simulink model "ES249A_MotAgCorrln"  (R2013b)
settings: Solver=FixedStepDiscrete  SolverMode=SingleTasking  StartTime=0.0  StopTime=1  FixedStep=0.002  RelTol=1e-3
undefined symbols (not defined in the file): FLTINJ_MOTAGCORRLN_MOTAGIDPTSIG, HALFREV_MOTREV_U0P16, MOTAGACORRLNST_CNT_U08, MotAgAMotAgBCorrln, MotAgAMotAgCCorrln, MOTAGBCORRLNST_CNT_U08, MotAgBMotAgCCorrln, MOTAGCCORRLNST_CNT_U08, MOTAGCORRLNERRTHD_MOTREVELEC_U0P16, MOTAGCORRLNNTCFAILSTEP_CNT_U16, MOTAGCORRLNNTCPASSSTEP_CNT_U16, MOTAGMAXSTALLCNTR_CNT_U08, MotAgMeclCorrlnSt, MotAgMeclIdptSig, NtcSts1, sigbuilder_block, SysGlbPrmMotPoleCnt
libraries: simulink x5
(part 2 of 4)

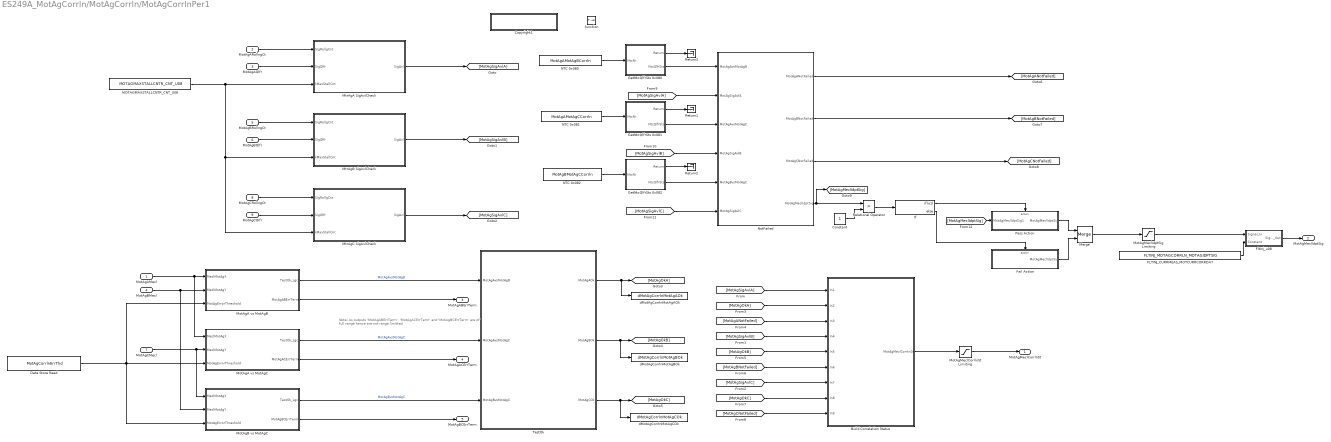
== system ES249A_MotAgCorrln/MotAgCorrln/MotAgCorrlnPer1 ==
  note: Note: As outputs 'MotAgABErrTerm', 'MotAgACErrTerm' and 'MotAgBCErrTerm'
      | are of full range hence are not range limitted
  MotAgAMecl : Inport  RequirementInfo={} %GIDa_0d510189_b4be_492d_be7e_b68d691b2df9
  MotAgARollngCt : Inport  RequirementInfo={} %GIDa_517e33a2_5a75_4f61_8f0f_573ac68cba90  Port=2
  MotAgAQlfr : Inport  RequirementInfo={} %GIDa_72867f98_7693_466f_aee4_0d6354195f1e  Port=3
  MotAgBMecl : Inport  RequirementInfo={} %GIDa_cfbccf8f_533e_4f37_986a_e6dac4ce98be  Port=4
  MotAgBRollngCt : Inport  RequirementInfo={} %GIDa_0bfa8ef6_2836_4615_abbf_8888cb320397  Port=5
  MotAgBQlfr : Inport  RequirementInfo={} %GIDa_efd6d5fa_412f_4474_a057_389b850e160a  Port=6
  MotAgCMecl : Inport  RequirementInfo={} %GIDa_b4666b4a_7a72_490a_9a26_ab5605674f7c  Port=7
  MotAgCRollngCt : Inport  RequirementInfo={} %GIDa_2a959797_a597_4b9a_b225_8bb1363b4372  Port=8
  MotAgCQlfr : Inport  RequirementInfo={} %GIDa_ae78480a_19b1_4014_b9a6_e3ccb226d53e  Port=9
  function : TriggerPort  RequirementInfo={'linktype_rmi_doors' '0000c47a (/E-STEER Core/SubSystem Specifications/Electrical Actuator/Control Module/FDD Module Requirements/EA4/ES249A_MotAgCorrln DRAFT)' '#ES249A_25' 'true' 'REQ: ES249A_25' '' ; 'linktype_rmi_doors' '0000c47a (/E-STEER Core/SubSystem Specifications/Electrical Actuator/Control Module/FDD Module Requirements/EA4/ES249A_MotAgCorrln DRAFT)' '#ES249A_76' 'true' 'REQ: ES249A_76' '' ; 'linktype_rmi_doors' '0000c47a (/E-STEER Core/SubSystem Specifications/Electrical Actuator/Control Module/FDD Module Requirements/EA4/ES249A_MotAgCorrln DRAFT)' '#ES249A_85' 'true' 'REQ: ES249A_85' '' } %GIDa_31db59e0_dbe3_46c8_b533_8d5601b81075  TriggerType=function-call
  Build Correlation Status : Subsystem  RequirementInfo={'linktype_rmi_doors' '0000c47a (/E-STEER Core/SubSystem Specifications/Electrical Actuator/Control Module/FDD Module Requirements/EA4/ES249A_MotAgCorrln DRAFT)' '#ES249A_90' 'true' 'REQ: ES249A_90' '' } %GIDa_aeadb70c_103d_495b_a56d_3da9c7a106e3
  Constant : Constant  RequirementInfo={'linktype_rmi_doors' '0000c47a (/E-STEER Core/SubSystem Specifications/Electrical Actuator/Control Module/FDD Module Requirements/EA4/ES249A_MotAgCorrln)' '#ES249A_110' 'true' 'REQ: ES249A_110' '' } %GIDa_5d96b250_1bd1_40e8_b31a_35961645f040  OutDataTypeStr=uint8
      settings: AttributesFormatString=%<OutDataTypeStr>
  Copyright1 : Subsystem  Description=|  RequirementInfo={} %GIDa_7b6edb4a_3f39_48e0_befb_44ef32e9295a  mask(Copyright Information){none=on}
      | Copyright info block.                                               
      |                                                                     
      | Place copyright information at the top of every subsystem in design.
      mask prompts: none "No parameters"
      mask help: Place copyright information at the top of every subsystem in design.
      mask Display:
      | NxtrConf = 'Nexteer Confidential';
      | 
      | sys = bdroot; %handle for the current model ("system")
      | first = get_param(sys,'Created');
      | if(isempty(first))
      |     first = datestr(now,'yyyy');
      | else
      |     first = first(end-3:end);  %year is last four digits
      | end
      | 
      | last = get_param(sys,'LastModifiedDate');
      | if isempty(last)
      |     last = datestr(now,'yyyy');
      | else
      |     last = last(end-3:end);
      | end
      | 
      | if strcmp(first,last)
      |     fprintf('%s\nCopyright  %s Nexteer',NxtrConf,first);
      | else
      |     fprintf('%s\n%s%s-%s Nexteer',NxtrConf,char(169),first,last);
      | end
  Data Store Read : DataStoreRead  DataStoreName=MotAgCorrlnErrThd
  FLTINJ_CURRMEAS_MOTCURRCORRDA7 : Constant  Value=FLTINJ_MOTAGCORRLN_MOTAGIDPTSIG
  "Fail Action " : Subsystem  RequirementInfo={'linktype_rmi_doors' '0000c47a (/E-STEER Core/SubSystem Specifications/Electrical Actuator/Control Module/FDD Module Requirements/EA4/ES249A_MotAgCorrln)' '#ES249A_110' 'true' 'REQ: ES249A_110' '' } %GIDa_4e6cbac2_25f9_4a00_a650_a831ef320943  TreatAsAtomicUnit=on
  "FltInj_u08 " : Subsystem  RequirementInfo={'linktype_rmi_doors' '0000c47a (/E-STEER Core/SubSystem Specifications/Electrical Actuator/Control Module/FDD Module Requirements/EA4/ES249A_MotAgCorrln)' '#ES249A_106' 'true' 'REQ: ES249A_106' '' } %GIDa_071c3215_62aa_4359_8caf_75f09dd6c30e  TreatAsAtomicUnit=on  VariantControl=FltInj_sim  mask(Fault_Injection){}
      mask help: Fault Injection is a simulation only block for EA3 programs.
  "GetNtcQlfrSts 0x080 " : Subsystem  RequirementInfo={'linktype_rmi_doors' '0000c47a (/E-STEER Core/SubSystem Specifications/Electrical Actuator/Control Module/FDD Module Requirements/EA4/ES249A_MotAgCorrln DRAFT)' '#ES249A_92' 'true' 'REQ: ES249A_92' '' ; 'linktype_rmi_doors' '0000c47a (/E-STEER Core/SubSystem Specifications/Electrical Actuator/Control Module/FDD Module Requirements/EA4/ES249A_MotAgCorrln DRAFT)' '#ES249A_96' 'true' 'REQ: ES249A_96' '' ; 'linktype_rmi_doors' '0000c47a (/E-STEER Core/SubSystem Specifications/Electrical Actuator/Control Module/FDD Module Requirements/EA4/ES249A_MotAgCorrln DRAFT)' '#ES249A_101' 'true' 'REQ: ES249A_101' '' ; 'linktype_rmi_doors' '0000c47a (/E-STEER Core/SubSystem Specifications/Electrical Actuator/Control Module/FDD Module Requirements/EA4/ES249A_MotAgCorrln DRAFT)' '#ES249A_102' 'true' 'REQ: ES249A_102' '' ; 'linktype_rmi_doors' '0000c47a (/E-STEER Core/SubSystem Specifications/Electrical Actuator/Control Module/FDD Module Requirements/EA4/ES249A_MotAgCorrln DRAFT)' '#ES249A_103' 'true' 'REQ: ES249A_103' '' ; 'linktype_rmi_doors' '0000c47a (/E-STEER Core/SubSystem Specifications/Electrical Actuator/Control Module/FDD Module Requirements/EA4/ES249A_MotAgCorrln DRAFT)' '#ES249A_97' 'true' 'REQ: ES249A_97' '' ; 'linktype_rmi_doors' '0000c47a (/E-STEER Core/SubSystem Specifications/Electrical Actuator/Control Module/FDD Module Requirements/EA4/ES249A_MotAgCorrln DRAFT)' '#ES249A_98' 'true' 'REQ: ES249A_98' '' ; 'linktype_rmi_doors' '0000c47a (/E-STEER Core/SubSystem Specifications/Electrical Actuator/Control Module/FDD Module Requirements/EA4/ES249A_MotAgCorrln DRAFT)' '#ES249A_96' 'true' 'REQ: ES249A_96' '' ; 'linktype_rmi_doors' '0000c47a (/E-STEER Core/SubSystem Specifications/Electrical Actuator/Control Module/FDD Module Requirements/EA4/ES249A_MotAgCorrln DRAFT)' '#ES249A_101' 'true' 'REQ: ES249A_101' '' ; 'linktype_rmi_doors' '0000c47a (/E-STEER Core/SubSystem Specifications/Electrical Actuator/Control Module/FDD Module Requirements/EA4/ES249A_MotAgCorrln DRAFT)' '#ES249A_102' 'true' 'REQ: ES249A_102' '' ; 'linktype_rmi_doors' '0000c47a (/E-STEER Core/SubSystem Specifications/Electrical Actuator/Control Module/FDD Module Requirements/EA4/ES249A_MotAgCorrln DRAFT)' '#ES249A_103' 'true' 'REQ: ES249A_103' '' ; 'linktype_rmi_doors' '0000c47a (/E-STEER Core/SubSystem Specifications/Electrical Actuator/Control Module/FDD Module Requirements/EA4/ES249A_MotAgCorrln DRAFT)' '#ES249A_97' 'true' 'REQ: ES249A_97' '' ; 'linktype_rmi_doors' '0000c47a (/E-STEER Core/SubSystem Specifications/Electrical Actuator/Control Module/FDD Module Requirements/EA4/ES249A_MotAgCorrln DRAFT)' '#ES249A_98' 'true' 'REQ: ES249A_98' '' ; 'linktype_rmi_doors' '0000c47a (/E-STEER Core/SubSystem Specifications/Electrical Actuator/Control Module/FDD Module Requirements/EA4/ES249A_MotAgCorrln DRAFT)' '#ES249A_104' 'true' 'REQ: ES249A_104' '' ; 'linktype_rmi_doors' '0000c47a (/E-STEER Core/SubSystem Specifications/Electrical Actuator/Control Module/FDD Module Requirements/EA4/ES249A_MotAgCorrln DRAFT)' '#ES249A_100' 'true' 'REQ: ES249A_100' '' } %GIDa_cf545445_441a_46fe_b236_5e2b4963b333
  GetNtcQlfrSts 0x081 : Subsystem  RequirementInfo={'linktype_rmi_doors' '0000c47a (/E-STEER Core/SubSystem Specifications/Electrical Actuator/Control Module/FDD Module Requirements/EA4/ES249A_MotAgCorrln DRAFT)' '#ES249A_92' 'true' 'REQ: ES249A_92' '' ; 'linktype_rmi_doors' '0000c47a (/E-STEER Core/SubSystem Specifications/Electrical Actuator/Control Module/FDD Module Requirements/EA4/ES249A_MotAgCorrln DRAFT)' '#ES249A_96' 'true' 'REQ: ES249A_96' '' ; 'linktype_rmi_doors' '0000c47a (/E-STEER Core/SubSystem Specifications/Electrical Actuator/Control Module/FDD Module Requirements/EA4/ES249A_MotAgCorrln DRAFT)' '#ES249A_101' 'true' 'REQ: ES249A_101' '' ; 'linktype_rmi_doors' '0000c47a (/E-STEER Core/SubSystem Specifications/Electrical Actuator/Control Module/FDD Module Requirements/EA4/ES249A_MotAgCorrln DRAFT)' '#ES249A_102' 'true' 'REQ: ES249A_102' '' ; 'linktype_rmi_doors' '0000c47a (/E-STEER Core/SubSystem Specifications/Electrical Actuator/Control Module/FDD Module Requirements/EA4/ES249A_MotAgCorrln DRAFT)' '#ES249A_103' 'true' 'REQ: ES249A_103' '' ; 'linktype_rmi_doors' '0000c47a (/E-STEER Core/SubSystem Specifications/Electrical Actuator/Control Module/FDD Module Requirements/EA4/ES249A_MotAgCorrln DRAFT)' '#ES249A_97' 'true' 'REQ: ES249A_97' '' ; 'linktype_rmi_doors' '0000c47a (/E-STEER Core/SubSystem Specifications/Electrical Actuator/Control Module/FDD Module Requirements/EA4/ES249A_MotAgCorrln DRAFT)' '#ES249A_98' 'true' 'REQ: ES249A_98' '' ; 'linktype_rmi_doors' '0000c47a (/E-STEER Core/SubSystem Specifications/Electrical Actuator/Control Module/FDD Module Requirements/EA4/ES249A_MotAgCorrln DRAFT)' '#ES249A_96' 'true' 'REQ: ES249A_96' '' ; 'linktype_rmi_doors' '0000c47a (/E-STEER Core/SubSystem Specifications/Electrical Actuator/Control Module/FDD Module Requirements/EA4/ES249A_MotAgCorrln DRAFT)' '#ES249A_101' 'true' 'REQ: ES249A_101' '' ; 'linktype_rmi_doors' '0000c47a (/E-STEER Core/SubSystem Specifications/Electrical Actuator/Control Module/FDD Module Requirements/EA4/ES249A_MotAgCorrln DRAFT)' '#ES249A_102' 'true' 'REQ: ES249A_102' '' ; 'linktype_rmi_doors' '0000c47a (/E-STEER Core/SubSystem Specifications/Electrical Actuator/Control Module/FDD Module Requirements/EA4/ES249A_MotAgCorrln DRAFT)' '#ES249A_103' 'true' 'REQ: ES249A_103' '' ; 'linktype_rmi_doors' '0000c47a (/E-STEER Core/SubSystem Specifications/Electrical Actuator/Control Module/FDD Module Requirements/EA4/ES249A_MotAgCorrln DRAFT)' '#ES249A_97' 'true' 'REQ: ES249A_97' '' ; 'linktype_rmi_doors' '0000c47a (/E-STEER Core/SubSystem Specifications/Electrical Actuator/Control Module/FDD Module Requirements/EA4/ES249A_MotAgCorrln DRAFT)' '#ES249A_98' 'true' 'REQ: ES249A_98' '' ; 'linktype_rmi_doors' '0000c47a (/E-STEER Core/SubSystem Specifications/Electrical Actuator/Control Module/FDD Module Requirements/EA4/ES249A_MotAgCorrln DRAFT)' '#ES249A_104' 'true' 'REQ: ES249A_104' '' ; 'linktype_rmi_doors' '0000c47a (/E-STEER Core/SubSystem Specifications/Electrical Actuator/Control Module/FDD Module Requirements/EA4/ES249A_MotAgCorrln DRAFT)' '#ES249A_100' 'true' 'REQ: ES249A_100' '' } %GIDa_4ee30c34_999a_4e6c_b4c1_ed28ed98d18e
  GetNtcQlfrSts 0x082 : Subsystem  RequirementInfo={'linktype_rmi_doors' '0000c47a (/E-STEER Core/SubSystem Specifications/Electrical Actuator/Control Module/FDD Module Requirements/EA4/ES249A_MotAgCorrln DRAFT)' '#ES249A_92' 'true' 'REQ: ES249A_92' '' ; 'linktype_rmi_doors' '0000c47a (/E-STEER Core/SubSystem Specifications/Electrical Actuator/Control Module/FDD Module Requirements/EA4/ES249A_MotAgCorrln DRAFT)' '#ES249A_96' 'true' 'REQ: ES249A_96' '' ; 'linktype_rmi_doors' '0000c47a (/E-STEER Core/SubSystem Specifications/Electrical Actuator/Control Module/FDD Module Requirements/EA4/ES249A_MotAgCorrln DRAFT)' '#ES249A_101' 'true' 'REQ: ES249A_101' '' ; 'linktype_rmi_doors' '0000c47a (/E-STEER Core/SubSystem Specifications/Electrical Actuator/Control Module/FDD Module Requirements/EA4/ES249A_MotAgCorrln DRAFT)' '#ES249A_102' 'true' 'REQ: ES249A_102' '' ; 'linktype_rmi_doors' '0000c47a (/E-STEER Core/SubSystem Specifications/Electrical Actuator/Control Module/FDD Module Requirements/EA4/ES249A_MotAgCorrln DRAFT)' '#ES249A_103' 'true' 'REQ: ES249A_103' '' ; 'linktype_rmi_doors' '0000c47a (/E-STEER Core/SubSystem Specifications/Electrical Actuator/Control Module/FDD Module Requirements/EA4/ES249A_MotAgCorrln DRAFT)' '#ES249A_97' 'true' 'REQ: ES249A_97' '' ; 'linktype_rmi_doors' '0000c47a (/E-STEER Core/SubSystem Specifications/Electrical Actuator/Control Module/FDD Module Requirements/EA4/ES249A_MotAgCorrln DRAFT)' '#ES249A_98' 'true' 'REQ: ES249A_98' '' ; 'linktype_rmi_doors' '0000c47a (/E-STEER Core/SubSystem Specifications/Electrical Actuator/Control Module/FDD Module Requirements/EA4/ES249A_MotAgCorrln DRAFT)' '#ES249A_96' 'true' 'REQ: ES249A_96' '' ; 'linktype_rmi_doors' '0000c47a (/E-STEER Core/SubSystem Specifications/Electrical Actuator/Control Module/FDD Module Requirements/EA4/ES249A_MotAgCorrln DRAFT)' '#ES249A_101' 'true' 'REQ: ES249A_101' '' ; 'linktype_rmi_doors' '0000c47a (/E-STEER Core/SubSystem Specifications/Electrical Actuator/Control Module/FDD Module Requirements/EA4/ES249A_MotAgCorrln DRAFT)' '#ES249A_102' 'true' 'REQ: ES249A_102' '' ; 'linktype_rmi_doors' '0000c47a (/E-STEER Core/SubSystem Specifications/Electrical Actuator/Control Module/FDD Module Requirements/EA4/ES249A_MotAgCorrln DRAFT)' '#ES249A_103' 'true' 'REQ: ES249A_103' '' ; 'linktype_rmi_doors' '0000c47a (/E-STEER Core/SubSystem Specifications/Electrical Actuator/Control Module/FDD Module Requirements/EA4/ES249A_MotAgCorrln DRAFT)' '#ES249A_97' 'true' 'REQ: ES249A_97' '' ; 'linktype_rmi_doors' '0000c47a (/E-STEER Core/SubSystem Specifications/Electrical Actuator/Control Module/FDD Module Requirements/EA4/ES249A_MotAgCorrln DRAFT)' '#ES249A_98' 'true' 'REQ: ES249A_98' '' ; 'linktype_rmi_doors' '0000c47a (/E-STEER Core/SubSystem Specifications/Electrical Actuator/Control Module/FDD Module Requirements/EA4/ES249A_MotAgCorrln DRAFT)' '#ES249A_104' 'true' 'REQ: ES249A_104' '' ; 'linktype_rmi_doors' '0000c47a (/E-STEER Core/SubSystem Specifications/Electrical Actuator/Control Module/FDD Module Requirements/EA4/ES249A_MotAgCorrln DRAFT)' '#ES249A_100' 'true' 'REQ: ES249A_100' '' } %GIDa_ec14c0cf_6648_43c4_b632_74a3cc3324ae
  If : If  RequirementInfo={'linktype_rmi_doors' '0000c47a (/E-STEER Core/SubSystem Specifications/Electrical Actuator/Control Module/FDD Module Requirements/EA4/ES249A_MotAgCorrln)' '#ES249A_110' 'true' 'REQ: ES249A_110' '' } %GIDa_46d2acb1_6297_426c_b0f5_297e7657a3b8  IfExpression=u1
  MOTAGMAXSTALLCNTR_CNT_U08 : Constant  RequirementInfo={} %GIDa_608cf4f3_c4d9_4650_bf98_959cd5939cb0  Value=MOTAGMAXSTALLCNTR_CNT_U08
  Merge : Merge
  MotAgA vs MotAgB : Subsystem  RequirementInfo={'linktype_rmi_doors' '0000c47a (/E-STEER Core/SubSystem Specifications/Electrical Actuator/Control Module/FDD Module Requirements/EA4/ES249A_MotAgCorrln DRAFT)' '#ES249A_91' 'true' 'REQ: ES249A_91' '' ; 'linktype_rmi_doors' '0000c47a (/E-STEER Core/SubSystem Specifications/Electrical Actuator/Control Module/FDD Module Requirements/EA4/ES249A_MotAgCorrln DRAFT)' '#ES249A_93' 'true' 'REQ: ES249A_93' '' ; 'linktype_rmi_doors' '0000c47a (/E-STEER Core/SubSystem Specifications/Electrical Actuator/Control Module/FDD Module Requirements/EA4/ES249A_MotAgCorrln DRAFT)' '#ES249A_22' 'true' 'REQ: ES249A_22' '' ; 'linktype_rmi_doors' '0000c47a (/E-STEER Core/SubSystem Specifications/Electrical Actuator/Control Module/FDD Module Requirements/EA4/ES249A_MotAgCorrln DRAFT)' '#ES249A_28' 'true' 'REQ: ES249A_28' '' ; 'linktype_rmi_doors' '0000c47a (/E-STEER Core/SubSystem Specifications/Electrical Actuator/Control Module/FDD Module Requirements/EA4/ES249A_MotAgCorrln DRAFT)' '#ES249A_107' 'true' 'REQ: ES249A_107' '' ; 'linktype_rmi_doors' '0000c47a (/E-STEER Core/SubSystem Specifications/Electrical Actuator/Control Module/FDD Module Requirements/EA4/ES249A_MotAgCorrln DRAFT)' '#ES249A_31' 'true' 'REQ: ES249A_31' '' } %GIDa_09b3f2ca_3360_4937_963b_0a8119aa0d87  TreatAsAtomicUnit=on
  MotAgA vs MotAgC : Subsystem  RequirementInfo={'linktype_rmi_doors' '0000c47a (/E-STEER Core/SubSystem Specifications/Electrical Actuator/Control Module/FDD Module Requirements/EA4/ES249A_MotAgCorrln DRAFT)' '#ES249A_91' 'true' 'REQ: ES249A_91' '' ; 'linktype_rmi_doors' '0000c47a (/E-STEER Core/SubSystem Specifications/Electrical Actuator/Control Module/FDD Module Requirements/EA4/ES249A_MotAgCorrln DRAFT)' '#ES249A_95' 'true' 'REQ: ES249A_95' '' ; 'linktype_rmi_doors' '0000c47a (/E-STEER Core/SubSystem Specifications/Electrical Actuator/Control Module/FDD Module Requirements/EA4/ES249A_MotAgCorrln DRAFT)' '#ES249A_74' 'true' 'REQ: ES249A_74' '' ; 'linktype_rmi_doors' '0000c47a (/E-STEER Core/SubSystem Specifications/Electrical Actuator/Control Module/FDD Module Requirements/EA4/ES249A_MotAgCorrln DRAFT)' '#ES249A_108' 'true' 'REQ: ES249A_108' '' ; 'linktype_rmi_doors' '0000c47a (/E-STEER Core/SubSystem Specifications/Electrical Actuator/Control Module/FDD Module Requirements/EA4/ES249A_MotAgCorrln DRAFT)' '#ES249A_78' 'true' 'REQ: ES249A_78' '' ; 'linktype_rmi_doors' '0000c47a (/E-STEER Core/SubSystem Specifications/Electrical Actuator/Control Module/FDD Module Requirements/EA4/ES249A_MotAgCorrln DRAFT)' '#ES249A_80' 'true' 'REQ: ES249A_80' '' } %GIDa_379fa372_061a_48aa_b00b_9e4c7a531b08  TreatAsAtomicUnit=on
  MotAgB vs MotAgC : Subsystem  RequirementInfo={'linktype_rmi_doors' '0000c47a (/E-STEER Core/SubSystem Specifications/Electrical Actuator/Control Module/FDD Module Requirements/EA4/ES249A_MotAgCorrln DRAFT)' '#ES249A_93' 'true' 'REQ: ES249A_93' '' ; 'linktype_rmi_doors' '0000c47a (/E-STEER Core/SubSystem Specifications/Electrical Actuator/Control Module/FDD Module Requirements/EA4/ES249A_MotAgCorrln DRAFT)' '#ES249A_95' 'true' 'REQ: ES249A_95' '' ; 'linktype_rmi_doors' '0000c47a (/E-STEER Core/SubSystem Specifications/Electrical Actuator/Control Module/FDD Module Requirements/EA4/ES249A_MotAgCorrln DRAFT)' '#ES249A_83' 'true' 'REQ: ES249A_83' '' ; 'linktype_rmi_doors' '0000c47a (/E-STEER Core/SubSystem Specifications/Electrical Actuator/Control Module/FDD Module Requirements/EA4/ES249A_MotAgCorrln DRAFT)' '#ES249A_109' 'true' 'REQ: ES249A_109' '' ; 'linktype_rmi_doors' '0000c47a (/E-STEER Core/SubSystem Specifications/Electrical Actuator/Control Module/FDD Module Requirements/EA4/ES249A_MotAgCorrln DRAFT)' '#ES249A_87' 'true' 'REQ: ES249A_87' '' } %GIDa_8857769b_037b_43ff_a793_06b6b60f6117  TreatAsAtomicUnit=on
  MotAgMeclCorrlnSt Limiting : Saturate  UpperLimit=MotAgMeclCorrlnSt.EngMax  LowerLimit=MotAgMeclCorrlnSt.EngMin
  MotAgMeclIdptSig Limiting : Saturate  UpperLimit=MotAgMeclIdptSig.EngMax  LowerLimit=MotAgMeclIdptSig.EngMin
  MtrAgA SigAvlCheck : Subsystem  RequirementInfo={'linktype_rmi_doors' '0000c47a (/E-STEER Core/SubSystem Specifications/Electrical Actuator/Control Module/FDD Module Requirements/EA4/ES249A_MotAgCorrln DRAFT)' '#ES249A_53' 'true' 'REQ: ES249A_53' '' } %GIDa_7d20d3b5_defb_4845_b48d_75bf829e2c25  TreatAsAtomicUnit=on
  MtrAgB SigAvlCheck : Subsystem  RequirementInfo={'linktype_rmi_doors' '0000c47a (/E-STEER Core/SubSystem Specifications/Electrical Actuator/Control Module/FDD Module Requirements/EA4/ES249A_MotAgCorrln DRAFT)' '#ES249A_53' 'true' 'REQ: ES249A_53' '' } %GIDa_e439906c_aead_491e_9a6c_f8170eb4d0a5  TreatAsAtomicUnit=on
  MtrAgC SigAvlCheck : Subsystem  RequirementInfo={'linktype_rmi_doors' '0000c47a (/E-STEER Core/SubSystem Specifications/Electrical Actuator/Control Module/FDD Module Requirements/EA4/ES249A_MotAgCorrln DRAFT)' '#ES249A_53' 'true' 'REQ: ES249A_53' '' } %GIDa_2a37cadc_ff60_4c7b_9a98_2579cbc5f3e2  TreatAsAtomicUnit=on
  NTC 0x080 : Constant  RequirementInfo={} %GIDa_0eea48c0_45e5_4398_a9be_a03239322b48  Value=MotAgAMotAgBCorrln
  NTC 0x081 : Constant  RequirementInfo={} %GIDa_7d4b9ece_1027_4692_9cf4_4e19d9bb5e2f  Value=MotAgAMotAgCCorrln
  NTC 0x082 : Constant  RequirementInfo={} %GIDa_e72174e6_0d5b_49ac_9dfc_99b58633dff6  Value=MotAgBMotAgCCorrln
  NotFailed : Truth Table  RequirementInfo={'linktype_rmi_doors' '0000c47a (/E-STEER Core/SubSystem Specifications/Electrical Actuator/Control Module/FDD Module Requirements/EA4/ES249A_MotAgCorrln DRAFT)' '#ES249A_96' 'true' 'REQ: ES249A_96' '' ; 'linktype_rmi_doors' '0000c47a (/E-STEER Core/SubSystem Specifications/Electrical Actuator/Control Module/FDD Module Requirements/EA4/ES249A_MotAgCorrln DRAFT)' '#ES249A_101' 'true' 'REQ: ES249A_101' '' ; 'linktype_rmi_doors' '0000c47a (/E-STEER Core/SubSystem Specifications/Electrical Actuator/Control Module/FDD Module Requirements/EA4/ES249A_MotAgCorrln DRAFT)' '#ES249A_102' 'true' 'REQ: ES249A_102' '' ; 'linktype_rmi_doors' '0000c47a (/E-STEER Core/SubSystem Specifications/Electrical Actuator/Control Module/FDD Module Requirements/EA4/ES249A_MotAgCorrln DRAFT)' '#ES249A_103' 'true' 'REQ: ES249A_103' '' ; 'linktype_rmi_doors' '0000c47a (/E-STEER Core/SubSystem Specifications/Electrical Actuator/Control Module/FDD Module Requirements/EA4/ES249A_MotAgCorrln DRAFT)' '#ES249A_97' 'true' 'REQ: ES249A_97' '' ; 'linktype_rmi_doors' '0000c47a (/E-STEER Core/SubSystem Specifications/Electrical Actuator/Control Module/FDD Module Requirements/EA4/ES249A_MotAgCorrln DRAFT)' '#ES249A_98' 'true' 'REQ: ES249A_98' '' ; 'linktype_rmi_doors' '0000c47a (/E-STEER Core/SubSystem Specifications/Electrical Actuator/Control Module/FDD Module Requirements/EA4/ES249A_MotAgCorrln DRAFT)' '#ES249A_96' 'true' 'REQ: ES249A_96' '' ; 'linktype_rmi_doors' '0000c47a (/E-STEER Core/SubSystem Specifications/Electrical Actuator/Control Module/FDD Module Requirements/EA4/ES249A_MotAgCorrln DRAFT)' '#ES249A_101' 'true' 'REQ: ES249A_101' '' ; 'linktype_rmi_doors' '0000c47a (/E-STEER Core/SubSystem Specifications/Electrical Actuator/Control Module/FDD Module Requirements/EA4/ES249A_MotAgCorrln DRAFT)' '#ES249A_102' 'true' 'REQ: ES249A_102' '' ; 'linktype_rmi_doors' '0000c47a (/E-STEER Core/SubSystem Specifications/Electrical Actuator/Control Module/FDD Module Requirements/EA4/ES249A_MotAgCorrln DRAFT)' '#ES249A_103' 'true' 'REQ: ES249A_103' '' ; 'linktype_rmi_doors' '0000c47a (/E-STEER Core/SubSystem Specifications/Electrical Actuator/Control Module/FDD Module Requirements/EA4/ES249A_MotAgCorrln DRAFT)' '#ES249A_97' 'true' 'REQ: ES249A_97' '' ; 'linktype_rmi_doors' '0000c47a (/E-STEER Core/SubSystem Specifications/Electrical Actuator/Control Module/FDD Module Requirements/EA4/ES249A_MotAgCorrln DRAFT)' '#ES249A_98' 'true' 'REQ: ES249A_98' '' ; 'linktype_rmi_doors' '0000c47a (/E-STEER Core/SubSystem Specifications/Electrical Actuator/Control Module/FDD Module Requirements/EA4/ES249A_MotAgCorrln DRAFT)' '#ES249A_104' 'true' 'REQ: ES249A_104' '' ; 'linktype_rmi_doors' '0000c47a (/E-STEER Core/SubSystem Specifications/Electrical Actuator/Control Module/FDD Module Requirements/EA4/ES249A_MotAgCorrln DRAFT)' '#ES249A_100' 'true' 'REQ: ES249A_100' '' } %GIDa_edf88c33_dc88_41ba_8594_5e52700b2291  TreatAsAtomicUnit=on
  "Pass Action " : Subsystem  RequirementInfo={'linktype_rmi_doors' '0000c47a (/E-STEER Core/SubSystem Specifications/Electrical Actuator/Control Module/FDD Module Requirements/EA4/ES249A_MotAgCorrln)' '#ES249A_110' 'true' 'REQ: ES249A_110' '' } %GIDa_df5c7e9b_ac59_4201_9380_8d9a04cafac6  TreatAsAtomicUnit=on
  Relational Operator : RelationalOperator  RequirementInfo={'linktype_rmi_doors' '0000c47a (/E-STEER Core/SubSystem Specifications/Electrical Actuator/Control Module/FDD Module Requirements/EA4/ES249A_MotAgCorrln)' '#ES249A_110' 'true' 'REQ: ES249A_110' '' } %GIDa_a4d93259_7d4d_44f4_8fc4_7847395214cb  Operator=>  OutDataTypeStr=boolean
  Return1 : Terminator
      settings: RequirementInfo={} %GIDa_75a67747_9ddb_4865_b03d_aec7815b8708
  Return2 : Terminator
      settings: RequirementInfo={} %GIDa_e5246cdf_b664_4da0_ab0c_012f931cd664
  Return3 : Terminator
      settings: RequirementInfo={} %GIDa_c9e19320_3f8d_4741_896e_f243d7830e4c
  TestOk : Truth Table  RequirementInfo={'linktype_rmi_doors' '0000c47a (/E-STEER Core/SubSystem Specifications/Electrical Actuator/Control Module/FDD Module Requirements/EA4/ES249A_MotAgCorrln DRAFT)' '#ES249A_91' 'true' 'REQ: ES249A_91' '' ; 'linktype_rmi_doors' '0000c47a (/E-STEER Core/SubSystem Specifications/Electrical Actuator/Control Module/FDD Module Requirements/EA4/ES249A_MotAgCorrln DRAFT)' '#ES249A_93' 'true' 'REQ: ES249A_93' '' ; 'linktype_rmi_doors' '0000c47a (/E-STEER Core/SubSystem Specifications/Electrical Actuator/Control Module/FDD Module Requirements/EA4/ES249A_MotAgCorrln DRAFT)' '#ES249A_95' 'true' 'REQ: ES249A_95' '' } %GIDa_1545c9fb_70a7_4c59_9a2b_e6ada44ad487  TreatAsAtomicUnit=on
  dMotAgCorrlnMotAgAOk : DataStoreWrite  RequirementInfo={} %GIDa_83af0017_845d_42a9_9791_0193bed95843  DataStoreName=dMotAgCorrlnMotAgAOk
  dMotAgCorrlnMotAgBOk : DataStoreWrite  RequirementInfo={} %GIDa_3532357d_cbc7_4e9f_92ff_534a59fa4be8  DataStoreName=dMotAgCorrlnMotAgBOk
  dMotAgCorrlnMotAgCOk : DataStoreWrite  RequirementInfo={} %GIDa_d29927e0_0edf_428a_9ee6_7108eda020e9  DataStoreName=dMotAgCorrlnMotAgCOk
  MotAgMeclCorrlnSt : Outport  RequirementInfo={} %GIDa_e94f5450_01bd_4b33_9e8b_f067b81cb070
  MotAgMeclIdptSig : Outport  RequirementInfo={} %GIDa_f44c3d14_99ac_4145_ace9_f5b4313ef171  Port=2  OutDataTypeStr=uint8
  MotAgABErrTerm : Outport  Port=3
  MotAgACErrTerm : Outport  Port=4
  MotAgBCErrTerm : Outport  Port=5
  wires:
  MOTAGMAXSTALLCNTR_CNT_U08/1 -> MtrAgC SigAvlCheck/3(kMaxStallCnt), MtrAgB SigAvlCheck/3(kMaxStallCnt), MtrAgA SigAvlCheck/3(kMaxStallCnt)
  MtrAgA SigAvlCheck/1(SigAvl) -> [MotAgSigAvlA]
  MtrAgC SigAvlCheck/1(SigAvl) -> [MotAgSigAvlC]
  MotAgA vs MotAgB/1(TestOk_Lgc) -> TestOk/1(MotAgAvsMotAgB)  "MotAgAvsMotAgB"
  MotAgA vs MotAgC/1(TestOk_Lgc) -> TestOk/2(MotAgAvsMotAgC)  "MotAgAvsMotAgC"
  Build Correlation Status/1(MotAgMeclCorrlnSt) -> MotAgMeclCorrlnSt Limiting/1
  MotAgB vs MotAgC/1(TestOk_Lgc) -> TestOk/3(MotAgBvsMotAgC)  "MotAgBvsMotAgC"
  "GetNtcQlfrSts 0x080 "/2(NtcQlfrSts) -> NotFailed/1(MotAgAvsMotAgB)
  NTC 0x080/1 -> "GetNtcQlfrSts 0x080 "/1(NtcNr)
  "GetNtcQlfrSts 0x080 "/1(Return) -> Return3/1
  GetNtcQlfrSts 0x081/2(NtcQlfrSts) -> NotFailed/3(MotAgAvsMotAgC)
  NTC 0x081/1 -> GetNtcQlfrSts 0x081/1(NtcNr)
  GetNtcQlfrSts 0x081/1(Return) -> Return1/1
  GetNtcQlfrSts 0x082/2(NtcQlfrSts) -> NotFailed/5(MotAgBvsMotAgC)
  NTC 0x082/1 -> GetNtcQlfrSts 0x082/1(NtcNr)
  GetNtcQlfrSts 0x082/1(Return) -> Return2/1
  MtrAgB SigAvlCheck/1(SigAvl) -> [MotAgSigAvlB]
  TestOk/1(MotAgAOk) -> dMotAgCorrlnMotAgAOk/1, [MotAgOkA]
  TestOk/2(MotAgBOk) -> dMotAgCorrlnMotAgBOk/1, [MotAgOkB]
  TestOk/3(MotAgCOk) -> dMotAgCorrlnMotAgCOk/1, [MotAgOkC]
  NotFailed/1(MotAgANotFailed) -> [MotAgANotFailed]
  NotFailed/2(MotAgBNotFailed) -> [MotAgBNotFailed]
  NotFailed/3(MotAgCNotFailed) -> [MotAgCNotFailed]
  [MotAgSigAvlA] -> Build Correlation Status/1(In1)
  [MotAgSigAvlB] -> Build Correlation Status/4(In4)
  [MotAgSigAvlC] -> Build Correlation Status/7(In7)
  [MotAgOkA] -> Build Correlation Status/2(In2)
  [MotAgANotFailed] -> Build Correlation Status/3(In3)
  [MotAgOkB] -> Build Correlation Status/5(In5)
  [MotAgBNotFailed] -> Build Correlation Status/6(In6)
  [MotAgOkC] -> Build Correlation Status/8(In8)
  [MotAgCNotFailed] -> Build Correlation Status/9(In9)
  Data Store Read/1 -> MotAgB vs MotAgC/3(MotAgErrorThreshold), MotAgA vs MotAgC/3(MotAgErrorThreshold), MotAgA vs MotAgB/3(MotAgErrorThreshold)
  MotAgMeclCorrlnSt Limiting/1 -> MotAgMeclCorrlnSt/1
  MotAgMeclIdptSig Limiting/1 -> "FltInj_u08 "/1(Signal_In)
  "FltInj_u08 "/1(Signal_Out) -> MotAgMeclIdptSig/1
  FLTINJ_CURRMEAS_MOTCURRCORRDA7/1 -> "FltInj_u08 "/2(Constant)
  MotAgBRollngCt/1 -> MtrAgB SigAvlCheck/1(SigRollgCnt)
  MotAgBQlfr/1 -> MtrAgB SigAvlCheck/2(SigQlfr)
  MotAgCRollngCt/1 -> MtrAgC SigAvlCheck/1(SigRollgCnt)
  MotAgCQlfr/1 -> MtrAgC SigAvlCheck/2(SigQlfr)
  MotAgAMecl/1 -> MotAgA vs MotAgC/1(MeclMotAgX), MotAgA vs MotAgB/1(MeclMotAgX)
  MotAgBMecl/1 -> MotAgB vs MotAgC/2(MeclMotAgY), MotAgA vs MotAgB/2(MeclMotAgY)
  MotAgARollngCt/1 -> MtrAgA SigAvlCheck/1(SigRollgCnt)
  MotAgAQlfr/1 -> MtrAgA SigAvlCheck/2(SigQlfr)
  MotAgCMecl/1 -> MotAgB vs MotAgC/1(MeclMotAgX), MotAgA vs MotAgC/2(MeclMotAgY)
  [MotAgSigAvlA] -> NotFailed/2(MotAgSigAvlA)
  [MotAgSigAvlB] -> NotFailed/4(MotAgSigAvlB)
  [MotAgSigAvlC] -> NotFailed/6(MotAgSigAvlC)
  NotFailed/4(MotAgMeclIdptSig) -> [MotAgMeclIdptSig], Relational Operator/1
  If/2 -> "Fail Action "/Action
  Merge/1 -> MotAgMeclIdptSig Limiting/1
  "Pass Action "/1(MotAgMeclIdptSig) -> Merge/1
  "Fail Action "/1(MotAgMeclIdptSig) -> Merge/2
  Relational Operator/1 -> If/1
  Constant/1 -> Relational Operator/2
  If/1 -> "Pass Action "/Action
  [MotAgMeclIdptSig] -> "Pass Action "/1(MotAgMeclIdptSig1)
  MotAgA vs MotAgB/2(MotAgABErrTerm) -> MotAgABErrTerm/1
  MotAgA vs MotAgC/2(MotAgACErrTerm) -> MotAgACErrTerm/1
  MotAgB vs MotAgC/2(MotAgBCErrTerm) -> MotAgBCErrTerm/1

== system ES249A_MotAgCorrln/SIMULATION ONLY/Signal Builder ==
  Demux : Demux  Tag=STV Demux  Outputs=9
  FromWs : FromWorkspace  Tag=STV FromWs  VariableName=tuvar  SampleTime=0
      SigBuilderData=|
      | common.afterFinalStr = 'Extrapolate'
      | common.sampleTime = 0
      | dataSet(1).timeRange = [0 10]
      | dataSet(1).name = 'MotAgAandBFail'
      | dataSet(2).timeRange = [0 10]
      | dataSet(2).name = 'FailAngleB'
      | dataSet(3).timeRange = [0 10]
      | dataSet(3).name = 'MotAgCFails'
      | dataSet(4).timeRange = [0 10]
      | dataSet(4).name = 'QualOnAFails2'
      | dataSet(5).timeRange = [0 10]
      | dataSet(5).name = 'FrozenCounterB'
      | dataSet(6).timeRange = [0 10]
      | dataSet(6).name = 'Rollover of signal misalignment'
      | dataSet(7).timeRange = [0 10]
      | dataSet(7).name = 'Rollover of signal misalignment in opposite direction'
      | dataSet(8).timeRange = [0 10]
      | dataSet(8).name = 'MotAgAandBFail1'
      | sbobj.Groups(1).Name = 'MotAgAandBFail'
      | sbobj.Groups(1).Signals(1).Name = 'Call_Init1'
      | sbobj.Groups(1).Signals(1).XData = [0 10]
      | sbobj.Groups(1).Signals(1).YData = [0 0]
      | sbobj.Groups(1).Signals(2).Name = 'Call_Per1'
      | sbobj.Groups(1).Signals(2).XData = [0 0.002 0.002 10]
      | sbobj.Groups(1).Signals(2).YData = [1 1 0 0]
      | sbobj.Groups(1).Signals(3).Name = 'MotAgA'
      | sbobj.Groups(1).Signals(3).XData = [0 0.020202020202 0.040404040404 0.0606060606061 0.0808080808081 0.10101010101 0.121212121212 0.141414141414 0.161616161616 0.181818181818 0.20202020202 0.222222222222 ... (496 elements, 1x496)]
      | sbobj.Groups(1).Signals(3).YData = [0.5 0.531711959828 0.563296226787 0.59462562218 0.625573993591 0.656016722849 0.68583122783 0.714897456045 0.74309836805 0.770320408728 0.796453964527 0.821393804843 ... (496 elements, 1x496)]
      | sbobj.Groups(1).Signals(4).Name = 'MotAgAQlfr'
      | sbobj.Groups(1).Signals(4).XData = [0 0.305 1 1 3.005 3.005 10]
      | sbobj.Groups(1).Signals(4).YData = [1 1 1 2 1 2 2]
      | sbobj.Groups(1).Signals(5).Name = 'MotAgB'
      | sbobj.Groups(1).Signals(5).XData = [0 0.020202020202 0.040404040404 0.0606060606061 0.0808080808081 0.10101010101 0.121212121212 0.141414141414 0.161616161616 0.181818181818 0.20202020202 0.222222222222 ... (500 elements, 1x500)]
      | sbobj.Groups(1).Signals(5).YData = [0.5 0.531711959828 0.563296226787 0.59462562218 0.625573993591 0.656016722849 0.68583122783 0.714897456045 0.74309836805 0.770320408728 0.796453964527 0.821393804843 ... (500 elements, 1x500)]
      | sbobj.Groups(1).Signals(6).Name = 'FailRollingCounterB'
      | sbobj.Groups(1).Signals(6).XData = [0 0.5 10]
      | sbobj.Groups(1).Signals(6).YData = [0 0 0]
      | sbobj.Groups(1).Signals(7).Name = 'MotAgBQlfr'
      | sbobj.Groups(1).Signals(7).XData = [0 10]
      | sbobj.Groups(1).Signals(7).YData = [1 1]
      | sbobj.Groups(1).Signals(8).Name = 'MotAgC'
      | sbobj.Groups(1).Signals(8).XData = [0 0.020202020202 0.040404040404 0.0606060606061 0.0808080808081 0.10101010101 0.121212121212 0.141414141414 0.161616161616 0.181818181818 0.20202020202 0.222222222222 ... (496 elements, 1x496)]
      | sbobj.Groups(1).Signals(8).YData = [0.5 0.531711959828 0.563296226787 0.59462562218 0.625573993591 0.656016722849 0.68583122783 0.714897456045 0.74309836805 0.770320408728 0.796453964527 0.821393804843 ... (496 elements, 1x496)]
      | sbobj.Groups(1).Signals(9).Name = 'MotAgCQlfr'
      | sbobj.Groups(1).Signals(9).XData = [0 10]
      | sbobj.Groups(1).Signals(9).YData = [1 1]
      | sbobj.Groups(2).Name = 'FailAngleB'
      | sbobj.Groups(2).Signals(1).Name = 'Call_Init1'
      | sbobj.Groups(2).Signals(1).XData = [0 10]
      | sbobj.Groups(2).Signals(1).YData = [0 0]
      | sbobj.Groups(2).Signals(2).Name = 'Call_Per1'
      | sbobj.Groups(2).Signals(2).XData = [0 0.002 0.002 10]
      | sbobj.Groups(2).Signals(2).YData = [1 1 0 0]
      | sbobj.Groups(2).Signals(3).Name = 'MotAgA'
      | sbobj.Groups(2).Signals(3).XData = [0 0.020202020202 0.040404040404 0.0606060606061 0.0808080808081 0.10101010101 0.121212121212 0.141414141414 0.161616161616 0.181818181818 0.20202020202 0.222222222222 ... (496 elements, 1x496)]
      | sbobj.Groups(2).Signals(3).YData = [0.5 0.531711959828 0.563296226787 0.59462562218 0.625573993591 0.656016722849 0.68583122783 0.714897456045 0.74309836805 0.770320408728 0.796453964527 0.821393804843 ... (496 elements, 1x496)]
      | sbobj.Groups(2).Signals(4).Name = 'MotAgAQlfr'
      | sbobj.Groups(2).Signals(4).XData = [0 0.305 1 1 3.005 3.005 10]
      | sbobj.Groups(2).Signals(4).YData = [1 1 1 2 1 2 2]
      | sbobj.Groups(2).Signals(5).Name = 'MotAgB'
      | sbobj.Groups(2).Signals(5).XData = [0 0.020202020202 0.040404040404 0.0606060606061 0.0808080808081 0.10101010101 0.121212121212 0.141414141414 0.161616161616 0.181818181818 0.20202020202 0.222222222222 ... (496 elements, 1x496)]
      | sbobj.Groups(2).Signals(5).YData = [0.5 0.531711959828 0.563296226787 0.59462562218 0.625573993591 0.656016722849 0.68583122783 0.714897456045 0.74309836805 0.770320408728 0.796453964527 0.821393804843 ... (496 elements, 1x496)]
      | sbobj.Groups(2).Signals(6).Name = 'FailRollingCounterB'
      | sbobj.Groups(2).Signals(6).XData = [0 0.5 10]
      | sbobj.Groups(2).Signals(6).YData = [0 0 0]
      | sbobj.Groups(2).Signals(7).Name = 'MotAgBQlfr'
      | sbobj.Groups(2).Signals(7).XData = [0 10]
      | sbobj.Groups(2).Signals(7).YData = [1 1]
      | sbobj.Groups(2).Signals(8).Name = 'MotAgC'
      | sbobj.Groups(2).Signals(8).XData = [0 0.020202020202 0.040404040404 0.0606060606061 0.0808080808081 0.10101010101 0.121212121212 0.141414141414 0.161616161616 0.181818181818 0.20202020202 0.222222222222 ... (496 elements, 1x496)]
      | sbobj.Groups(2).Signals(8).YData = [0.5 0.531711959828 0.563296226787 0.59462562218 0.625573993591 0.656016722849 0.68583122783 0.714897456045 0.74309836805 0.770320408728 0.796453964527 0.821393804843 ... (496 elements, 1x496)]
      | sbobj.Groups(2).Signals(9).Name = 'MotAgCQlfr'
      | sbobj.Groups(2).Signals(9).XData = [0 10]
      | sbobj.Groups(2).Signals(9).YData = [1 1]
      | sbobj.Groups(3).Name = 'MotAgCFails'
      | sbobj.Groups(3).Signals(1).Name = 'Call_Init1'
      | sbobj.Groups(3).Signals(1).XData = [0 10]
      | sbobj.Groups(3).Signals(1).YData = [0 0]
      | sbobj.Groups(3).Signals(2).Name = 'Call_Per1'
      | sbobj.Groups(3).Signals(2).XData = [0 0.002 0.002 10]
      | sbobj.Groups(3).Signals(2).YData = [1 1 0 0]
      | sbobj.Groups(3).Signals(3).Name = 'MotAgA'
      | sbobj.Groups(3).Signals(3).XData = [0 0.020202020202 0.040404040404 0.0606060606061 0.0808080808081 0.10101010101 0.121212121212 0.141414141414 0.161616161616 0.181818181818 0.20202020202 0.222222222222 ... (496 elements, 1x496)]
      | sbobj.Groups(3).Signals(3).YData = [0.5 0.531711959828 0.563296226787 0.59462562218 0.625573993591 0.656016722849 0.68583122783 0.714897456045 0.74309836805 0.770320408728 0.796453964527 0.821393804843 ... (496 elements, 1x496)]
      | sbobj.Groups(3).Signals(4).Name = 'MotAgAQlfr'
      | sbobj.Groups(3).Signals(4).XData = [0 0.305 1 1 3.005 3.005 10]
      | sbobj.Groups(3).Signals(4).YData = [1 1 1 2 1 2 2]
      | sbobj.Groups(3).Signals(5).Name = 'MotAgB'
      | sbobj.Groups(3).Signals(5).XData = [0 0.020202020202 0.040404040404 0.0606060606061 0.0808080808081 0.10101010101 0.121212121212 0.141414141414 0.161616161616 0.181818181818 0.20202020202 0.222222222222 ... (496 elements, 1x496)]
      | sbobj.Groups(3).Signals(5).YData = [0.5 0.531711959828 0.563296226787 0.59462562218 0.625573993591 0.656016722849 0.68583122783 0.714897456045 0.74309836805 0.770320408728 0.796453964527 0.821393804843 ... (496 elements, 1x496)]
      | sbobj.Groups(3).Signals(6).Name = 'FailRollingCounterB'
      | sbobj.Groups(3).Signals(6).XData = [0 0.5 10]
      | sbobj.Groups(3).Signals(6).YData = [0 0 0]
      | sbobj.Groups(3).Signals(7).Name = 'MotAgBQlfr'
      | sbobj.Groups(3).Signals(7).XData = [0 10]
      | sbobj.Groups(3).Signals(7).YData = [1 1]
      | sbobj.Groups(3).Signals(8).Name = 'MotAgC'
      | sbobj.Groups(3).Signals(8).XData = [0 0.020202020202 0.040404040404 0.0606060606061 0.0808080808081 0.10101010101 0.121212121212 0.141414141414 0.161616161616 0.181818181818 0.20202020202 0.222222222222 ... (496 elements, 1x496)]
      | sbobj.Groups(3).Signals(8).YData = [0.5 0.531711959828 0.563296226787 0.59462562218 0.625573993591 0.656016722849 0.68583122783 0.714897456045 0.74309836805 0.770320408728 0.796453964527 0.821393804843 ... (496 elements, 1x496)]
      | sbobj.Groups(3).Signals(9).Name = 'MotAgCQlfr'
      | sbobj.Groups(3).Signals(9).XData = [0 10]
      | sbobj.Groups(3).Signals(9).YData = [1 1]
      | sbobj.Groups(4).Name = 'QualOnAFails2'
      | sbobj.Groups(4).Signals(1).Name = 'Call_Init1'
      | sbobj.Groups(4).Signals(1).XData = [0 10]
      | sbobj.Groups(4).Signals(1).YData = [0 0]
      | sbobj.Groups(4).Signals(2).Name = 'Call_Per1'
      | sbobj.Groups(4).Signals(2).XData = [0 0.002 0.002 10]
      | sbobj.Groups(4).Signals(2).YData = [1 1 0 0]
      | sbobj.Groups(4).Signals(3).Name = 'MotAgA'
      | sbobj.Groups(4).Signals(3).XData = [0 0.020202020202 0.040404040404 0.0606060606061 0.0808080808081 0.10101010101 0.121212121212 0.141414141414 0.161616161616 0.181818181818 0.20202020202 0.222222222222 ... (496 elements, 1x496)]
      | sbobj.Groups(4).Signals(3).YData = [0.5 0.531711959828 0.563296226787 0.59462562218 0.625573993591 0.656016722849 0.68583122783 0.714897456045 0.74309836805 0.770320408728 0.796453964527 0.821393804843 ... (496 elements, 1x496)]
      | sbobj.Groups(4).Signals(4).Name = 'MotAgAQlfr'
      | sbobj.Groups(4).Signals(4).XData = [0 0.305 0.305 1 3.005 3.005 10]
      | sbobj.Groups(4).Signals(4).YData = [1 1 2 2 1 2 2]
      | sbobj.Groups(4).Signals(5).Name = 'MotAgB'
      | sbobj.Groups(4).Signals(5).XData = [0 0.020202020202 0.040404040404 0.0606060606061 0.0808080808081 0.10101010101 0.121212121212 0.141414141414 0.161616161616 0.181818181818 0.20202020202 0.222222222222 ... (496 elements, 1x496)]
      | sbobj.Groups(4).Signals(5).YData = [0.5 0.531711959828 0.563296226787 0.59462562218 0.625573993591 0.656016722849 0.68583122783 0.714897456045 0.74309836805 0.770320408728 0.796453964527 0.821393804843 ... (496 elements, 1x496)]
      | sbobj.Groups(4).Signals(6).Name = 'FailRollingCounterB'
      | sbobj.Groups(4).Signals(6).XData = [0 0.5 10]
      | sbobj.Groups(4).Signals(6).YData = [0 0 0]
      | sbobj.Groups(4).Signals(7).Name = 'MotAgBQlfr'
      | sbobj.Groups(4).Signals(7).XData = [0 10]
      | sbobj.Groups(4).Signals(7).YData = [1 1]
      | sbobj.Groups(4).Signals(8).Name = 'MotAgC'
      | sbobj.Groups(4).Signals(8).XData = [0 0.020202020202 0.040404040404 0.0606060606061 0.0808080808081 0.10101010101 0.121212121212 0.141414141414 0.161616161616 0.181818181818 0.20202020202 0.222222222222 ... (496 elements, 1x496)]
      | sbobj.Groups(4).Signals(8).YData = [0.5 0.531711959828 0.563296226787 0.59462562218 0.625573993591 0.656016722849 0.68583122783 0.714897456045 0.74309836805 0.770320408728 0.796453964527 0.821393804843 ... (496 elements, 1x496)]
      | sbobj.Groups(4).Signals(9).Name = 'MotAgCQlfr'
      | sbobj.Groups(4).Signals(9).XData = [0 10]
      | sbobj.Groups(4).Signals(9).YData = [1 1]
      | sbobj.Groups(5).Name = 'FrozenCounterB'
      | sbobj.Groups(5).Signals(1).Name = 'Call_Init1'
      | sbobj.Groups(5).Signals(1).XData = [0 10]
      | sbobj.Groups(5).Signals(1).YData = [0 0]
      | sbobj.Groups(5).Signals(2).Name = 'Call_Per1'
      | sbobj.Groups(5).Signals(2).XData = [0 0.002 0.002 10]
      | sbobj.Groups(5).Signals(2).YData = [1 1 0 0]
      | sbobj.Groups(5).Signals(3).Name = 'MotAgA'
      | sbobj.Groups(5).Signals(3).XData = [0 0.020202020202 0.040404040404 0.0606060606061 0.0808080808081 0.10101010101 0.121212121212 0.141414141414 0.161616161616 0.181818181818 0.20202020202 0.222222222222 ... (496 elements, 1x496)]
      | sbobj.Groups(5).Signals(3).YData = [0.5 0.531711959828 0.563296226787 0.59462562218 0.625573993591 0.656016722849 0.68583122783 0.714897456045 0.74309836805 0.770320408728 0.796453964527 0.821393804843 ... (496 elements, 1x496)]
      | sbobj.Groups(5).Signals(4).Name = 'MotAgAQlfr'
      | sbobj.Groups(5).Signals(4).XData = [0 0.305 1 1 3.005 3.005 10]
      | sbobj.Groups(5).Signals(4).YData = [1 1 1 2 1 2 2]
      | sbobj.Groups(5).Signals(5).Name = 'MotAgB'
      | sbobj.Groups(5).Signals(5).XData = [0 0.020202020202 0.040404040404 0.0606060606061 0.0808080808081 0.10101010101 0.121212121212 0.141414141414 0.161616161616 0.181818181818 0.20202020202 0.222222222222 ... (496 elements, 1x496)]
      | sbobj.Groups(5).Signals(5).YData = [0.5 0.531711959828 0.563296226787 0.59462562218 0.625573993591 0.656016722849 0.68583122783 0.714897456045 0.74309836805 0.770320408728 0.796453964527 0.821393804843 ... (496 elements, 1x496)]
      | sbobj.Groups(5).Signals(6).Name = 'FailRollingCounterB'
      | sbobj.Groups(5).Signals(6).XData = [0 0.138 0.138 0.4 0.4 10]
      | sbobj.Groups(5).Signals(6).YData = [0 0 1 1 0 1]
      | sbobj.Groups(5).Signals(7).Name = 'MotAgBQlfr'
      | sbobj.Groups(5).Signals(7).XData = [0 10]
      | sbobj.Groups(5).Signals(7).YData = [1 1]
      | sbobj.Groups(5).Signals(8).Name = 'MotAgC'
      | sbobj.Groups(5).Signals(8).XData = [0 0.020202020202 0.040404040404 0.0606060606061 0.0808080808081 0.10101010101 0.121212121212 0.141414141414 0.161616161616 0.181818181818 0.20202020202 0.222222222222 ... (496 elements, 1x496)]
      | sbobj.Groups(5).Signals(8).YData = [0.5 0.531711959828 0.563296226787 0.59462562218 0.625573993591 0.656016722849 0.68583122783 0.714897456045 0.74309836805 0.770320408728 0.796453964527 0.821393804843 ... (496 elements, 1x496)]
      | sbobj.Groups(5).Signals(9).Name = 'MotAgCQlfr'
      | sbobj.Groups(5).Signals(9).XData = [0 10]
      | sbobj.Groups(5).Signals(9).YData = [1 1]
      | sbobj.Groups(6).Name = 'Rollover of signal misalignment'
      | sbobj.Groups(6).Signals(1).Name = 'Call_Init1'
      | sbobj.Groups(6).Signals(1).XData = [0 0.002 0.002 10]
      | sbobj.Groups(6).Signals(1).YData = [1 1 0 0]
      | sbobj.Groups(6).Signals(2).Name = 'Call_Per1'
      | sbobj.Groups(6).Signals(2).XData = [0 0.004 0.004 10]
      | sbobj.Groups(6).Signals(2).YData = [0 0 1 1]
      | sbobj.Groups(6).Signals(3).Name = 'MotAgA'
      | sbobj.Groups(6).Signals(3).XData = [0 0.4 0.4 0.7 0.7 10]
      | sbobj.Groups(6).Signals(3).YData = [0 1 0 1 0 0]
      | sbobj.Groups(6).Signals(4).Name = 'MotAgAQlfr'
      | sbobj.Groups(6).Signals(4).XData = [0 0.305 1 1 3.005 3.005 10]
      | sbobj.Groups(6).Signals(4).YData = [1 1 1 2 1 2 2]
      | sbobj.Groups(6).Signals(5).Name = 'MotAgB'
      | sbobj.Groups(6).Signals(5).XData = [0 0.392 0.392 0.707 0.707 10]
      | sbobj.Groups(6).Signals(5).YData = [0 1 0 1 0 0]
      | sbobj.Groups(6).Signals(6).Name = 'FailRollingCounterB'
      | sbobj.Groups(6).Signals(6).XData = [0 0.138 0.4 10]
      | sbobj.Groups(6).Signals(6).YData = [0 0 0 1]
      | sbobj.Groups(6).Signals(7).Name = 'MotAgBQlfr'
      | sbobj.Groups(6).Signals(7).XData = [0 10]
      | sbobj.Groups(6).Signals(7).YData = [1 1]
      | sbobj.Groups(6).Signals(8).Name = 'MotAgC'
      | sbobj.Groups(6).Signals(8).XData = [0 0.409 0.409 0.691 0.691 10]
      | sbobj.Groups(6).Signals(8).YData = [0 1 0 1 0 0]
      | sbobj.Groups(6).Signals(9).Name = 'MotAgCQlfr'
      | sbobj.Groups(6).Signals(9).XData = [0 10]
      | sbobj.Groups(6).Signals(9).YData = [1 1]
      | sbobj.Groups(7).Name = 'Rollover of signal misalignment in opposite direction'
      | sbobj.Groups(7).Signals(1).Name = 'Call_Init1'
      | sbobj.Groups(7).Signals(1).XData = [0 0.002 0.002 10]
      | sbobj.Groups(7).Signals(1).YData = [1 1 0 0]
      | sbobj.Groups(7).Signals(2).Name = 'Call_Per1'
      | sbobj.Groups(7).Signals(2).XData = [0 0.004 0.004 10]
      | sbobj.Groups(7).Signals(2).YData = [0 0 1 1]
      | sbobj.Groups(7).Signals(3).Name = 'MotAgA'
      | sbobj.Groups(7).Signals(3).XData = [0 0.4 0.4 0.7 0.7 1 10]
      | sbobj.Groups(7).Signals(3).YData = [1 0 1 0 1 0 0]
      | sbobj.Groups(7).Signals(4).Name = 'MotAgAQlfr'
      | sbobj.Groups(7).Signals(4).XData = [0 0.305 1 1 3.005 3.005 10]
      | sbobj.Groups(7).Signals(4).YData = [1 1 1 2 1 2 2]
      | sbobj.Groups(7).Signals(5).Name = 'MotAgB'
      | sbobj.Groups(7).Signals(5).XData = [0 0.392 0.392 0.707 0.707 1 10]
      | sbobj.Groups(7).Signals(5).YData = [1 0 1 0 1 0 0]
      | sbobj.Groups(7).Signals(6).Name = 'FailRollingCounterB'
      | sbobj.Groups(7).Signals(6).XData = [0 0.138 0.4 10]
      | sbobj.Groups(7).Signals(6).YData = [0 0 0 1]
      | sbobj.Groups(7).Signals(7).Name = 'MotAgBQlfr'
      | sbobj.Groups(7).Signals(7).XData = [0 10]
      | sbobj.Groups(7).Signals(7).YData = [1 1]
      | sbobj.Groups(7).Signals(8).Name = 'MotAgC'
      | sbobj.Groups(7).Signals(8).XData = [0 0.409 0.409 0.691 0.691 1 10]
      | sbobj.Groups(7).Signals(8).YData = [1 0 1 0 1 0 0]
      | sbobj.Groups(7).Signals(9).Name = 'MotAgCQlfr'
      | sbobj.Groups(7).Signals(9).XData = [0 10]
      | sbobj.Groups(7).Signals(9).YData = [1 1]
      | sbobj.Groups(8).Name = 'MotAgAandBFail1'
      | sbobj.Groups(8).Signals(1).Name = 'Call_Init1'
      | sbobj.Groups(8).Signals(1).XData = [0 10]
      | sbobj.Groups(8).Signals(1).YData = [0 0]
      | sbobj.Groups(8).Signals(2).Name = 'Call_Per1'
      | sbobj.Groups(8).Signals(2).XData = [0 0.002 0.002 10]
      | sbobj.Groups(8).Signals(2).YData = [1 1 0 0]
      | sbobj.Groups(8).Signals(3).Name = 'MotAgA'
      | sbobj.Groups(8).Signals(3).XData = [0 0.020202020202 0.040404040404 0.0606060606061 0.0808080808081 0.10101010101 0.121212121212 0.141414141414 0.161616161616 0.181818181818 0.20202020202 0.222222222222 ... (496 elements, 1x496)]
      | sbobj.Groups(8).Signals(3).YData = [0.5 0.531711959828 0.563296226787 0.59462562218 0.625573993591 0.656016722849 0.68583122783 0.714897456045 0.74309836805 0.770320408728 0.796453964527 0.821393804843 ... (496 elements, 1x496)]
      | sbobj.Groups(8).Signals(4).Name = 'MotAgAQlfr'
      | sbobj.Groups(8).Signals(4).XData = [0 0.305 1 1 3.005 3.005 10]
      | sbobj.Groups(8).Signals(4).YData = [1 1 1 2 1 2 2]
      | sbobj.Groups(8).Signals(5).Name = 'MotAgB'
      | sbobj.Groups(8).Signals(5).XData = [0 0.020202020202 0.040404040404 0.0606060606061 0.0808080808081 0.10101010101 0.121212121212 0.141414141414 0.161616161616 0.181818181818 0.20202020202 0.222222222222 ... (500 elements, 1x500)]
      | sbobj.Groups(8).Signals(5).YData = [0.5 0.531711959828 0.563296226787 0.59462562218 0.625573993591 0.656016722849 0.68583122783 0.714897456045 0.74309836805 0.770320408728 0.796453964527 0.821393804843 ... (500 elements, 1x500)]
      | sbobj.Groups(8).Signals(6).Name = 'FailRollingCounterB'
      | sbobj.Groups(8).Signals(6).XData = [0 0.5 10]
      | sbobj.Groups(8).Signals(6).YData = [0 0 0]
      | sbobj.Groups(8).Signals(7).Name = 'MotAgBQlfr'
      | sbobj.Groups(8).Signals(7).XData = [0 10]
      | sbobj.Groups(8).Signals(7).YData = [1 1]
      | sbobj.Groups(8).Signals(8).Name = 'MotAgC'
      | sbobj.Groups(8).Signals(8).XData = [0 0.020202020202 0.040404040404 0.0606060606061 0.0808080808081 0.10101010101 0.121212121212 0.141414141414 0.161616161616 0.181818181818 0.20202020202 0.222222222222 ... (496 elements, 1x496)]
      | sbobj.Groups(8).Signals(8).YData = [0.5 0.531711959828 0.563296226787 0.59462562218 0.625573993591 0.656016722849 0.68583122783 0.714897456045 0.74309836805 0.770320408728 0.796453964527 0.821393804843 ... (496 elements, 1x496)]
      | sbobj.Groups(8).Signals(9).Name = 'MotAgCQlfr'
      | sbobj.Groups(8).Signals(9).XData = [0 10]
      | sbobj.Groups(8).Signals(9).YData = [1 1]
  Call_Init1 : Outport  Tag=STV Outport
  Call_Per1 : Outport  Tag=STV Outport  Port=2
  MotAgA : Outport  Tag=STV Outport  Port=3
  MotAgAQlfr : Outport  Tag=STV Outport  Port=4
  MotAgB : Outport  Tag=STV Outport  Port=5
  FailRollingCounterB : Outport  Tag=STV Outport  Port=6
  MotAgBQlfr : Outport  Tag=STV Outport  Port=7
  MotAgC : Outport  Tag=STV Outport  Port=8
  MotAgCQlfr : Outport  Tag=STV Outport  Port=9
  wires:
  FromWs/1 -> Demux/1
  Demux/1 -> Call_Init1/1
  Demux/2 -> Call_Per1/1
  Demux/3 -> MotAgA/1
  Demux/4 -> MotAgAQlfr/1
  Demux/5 -> MotAgB/1
  Demux/6 -> FailRollingCounterB/1
  Demux/7 -> MotAgBQlfr/1
  Demux/8 -> MotAgC/1
  Demux/9 -> MotAgCQlfr/1

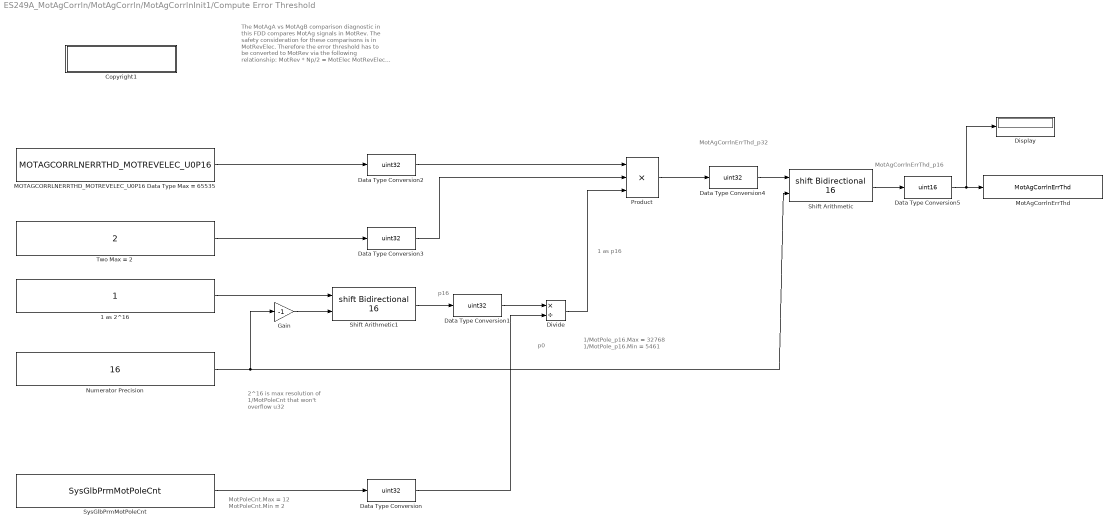
== system ES249A_MotAgCorrln/MotAgCorrln/MotAgCorrlnInit1/Compute Error Threshold ==
  note: MotAgCorrlnErrThd_p32
  note: p16
  note: p0
  note: 2^16 is max resolution
      | of 1/MotPoleCnt that won't
      | overflow u32
  note: MotPoleCnt.Max = 12
      | MotPoleCnt.Min = 2
  note: The MotAgA vs MotAgB comparison diagnostic
      | in this FDD compares MotAg signals in MotRev.
      | The safety consideration for these comparisons
      | is in MotRevElec.  Therefore the error threshold
      | has to be converted to MotRev via the following
      | relationship:
      |
      | MotRev * Np/2 = MotElec
      | MotRevElec * 2/Np = MotRev
  note: 1/MotPole_p16.Max = 32768
      | 1/MotPole_p16.Min = 5461
  note: 1 as p16
  note: MotAgCorrlnErrThd_p16
  1 as 2^16 : Constant  OutDataTypeStr=uint32
  Copyright1 : Subsystem  Description=|  RequirementInfo={} %GIDa_bacad073_da82_4802_ac19_55ca73cc7f3d  mask(Copyright Information){none=on}
      | Copyright info block.                                               
      |                                                                     
      | Place copyright information at the top of every subsystem in design.
      mask prompts: none "No parameters"
      mask help: Place copyright information at the top of every subsystem in design.
      mask Display:
      | NxtrConf = 'Nexteer Confidential';
      | 
      | sys = bdroot; %handle for the current model ("system")
      | first = get_param(sys,'Created');
      | if(isempty(first))
      |     first = datestr(now,'yyyy');
      | else
      |     first = first(end-3:end);  %year is last four digits
      | end
      | 
      | last = get_param(sys,'LastModifiedDate');
      | if isempty(last)
      |     last = datestr(now,'yyyy');
      | else
      |     last = last(end-3:end);
      | end
      | 
      | if strcmp(first,last)
      |     fprintf('%s\nCopyright  %s Nexteer',NxtrConf,first);
      | else
      |     fprintf('%s\n%s%s-%s Nexteer',NxtrConf,char(169),first,last);
      | end
  Data Type Conversion{,1..4} (5 alike) : DataTypeConversion  OutDataTypeStr=uint32
  Data Type Conversion5 : DataTypeConversion  OutDataTypeStr=uint16
  Display : Display
  Divide : Product  Inputs=*/
  Gain : Gain  Gain=-1  OutDataTypeStr=int8
  MOTAGCORRLNERRTHD_MOTREVELEC_U0P16 Data Type Max = 65535 : Constant  Value=MOTAGCORRLNERRTHD_MOTREVELEC_U0P16
  MotAgCorrlnErrThd : DataStoreWrite  DataStoreName=MotAgCorrlnErrThd
  Numerator Precision : Constant  Value=16  OutDataTypeStr=int8
  Product : Product  Inputs=3
  Shift Arithmetic : ArithShift  BitShiftNumberSource=Input port  BitShiftNumber=16
      settings: InputPortMap=u0,p1
  Shift Arithmetic1 : ArithShift  BitShiftNumberSource=Input port  BitShiftNumber=16
      settings: InputPortMap=u0,p1
  SysGlbPrmMotPoleCnt : Constant  Value=SysGlbPrmMotPoleCnt
  Two Max = 2 : Constant  Value=2  OutDataTypeStr=uint32
  wires:
  SysGlbPrmMotPoleCnt/1 -> Data Type Conversion/1
  1 as 2^16/1 -> Shift Arithmetic1/1
  Shift Arithmetic1/1 -> Data Type Conversion1/1
  Data Type Conversion/1 -> Divide/2
  MOTAGCORRLNERRTHD_MOTREVELEC_U0P16 Data Type Max = 65535/1 -> Data Type Conversion2/1
  Two Max = 2/1 -> Data Type Conversion3/1
  Divide/1 -> Product/3
  Product/1 -> Data Type Conversion4/1
  Data Type Conversion3/1 -> Product/2
  Data Type Conversion2/1 -> Product/1
  Data Type Conversion5/1 -> Display/1, MotAgCorrlnErrThd/1
  Data Type Conversion4/1 -> Shift Arithmetic/1
  Shift Arithmetic/1 -> Data Type Conversion5/1
  Numerator Precision/1 -> Gain/1, Shift Arithmetic/2
  Gain/1 -> Shift Arithmetic1/2
  Data Type Conversion1/1 -> Divide/1

== system ES249A_MotAgCorrln/MotAgCorrln/MotAgCorrlnInit1/Copyright1 ==

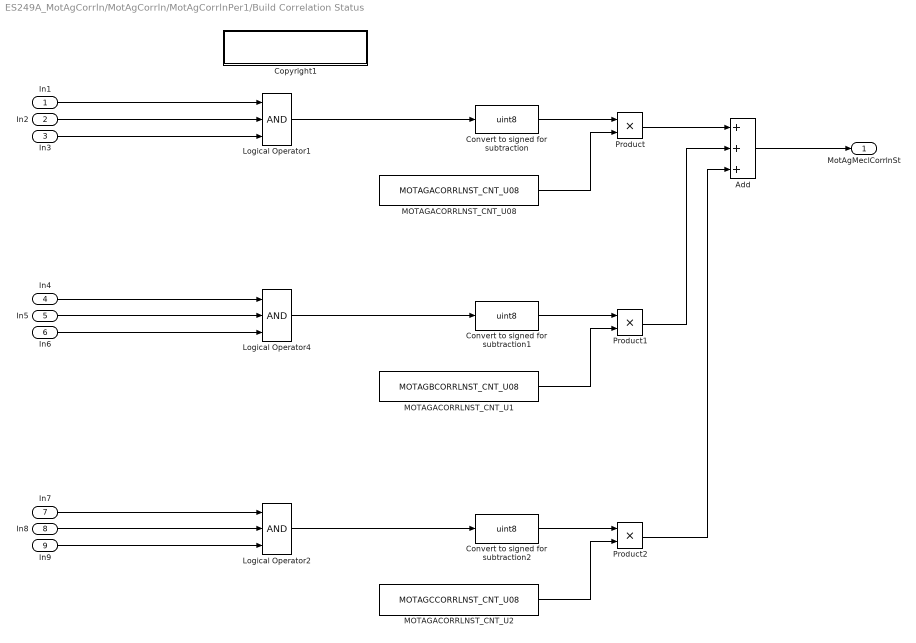
== system ES249A_MotAgCorrln/MotAgCorrln/MotAgCorrlnPer1/Build Correlation Status ==
  In1 : Inport  RequirementInfo={} %GIDa_cd681b8f_c92f_4b50_9e7d_92bc6119e047
  In2 : Inport  RequirementInfo={} %GIDa_f44a19ed_8f72_4e41_8f9f_0f92daa4024c  Port=2
  In3 : Inport  RequirementInfo={} %GIDa_9e5ac56c_3b1e_4699_a554_d66f898e46b8  Port=3
  In4 : Inport  RequirementInfo={} %GIDa_aebf03a5_3336_4a5f_8afb_527468548636  Port=4
  In5 : Inport  RequirementInfo={} %GIDa_7cfe586d_92e7_4163_b0bd_3ba9599ddb81  Port=5
  In6 : Inport  RequirementInfo={} %GIDa_de8aba0c_2029_44e3_a534_d103dd50ad22  Port=6
  In7 : Inport  RequirementInfo={} %GIDa_db3680f5_566b_40a5_b9ea_5ca3f2495fa5  Port=7
  In8 : Inport  RequirementInfo={} %GIDa_91ab37b8_a752_42f4_8db6_e934e5a68539  Port=8
  In9 : Inport  RequirementInfo={} %GIDa_1aad1152_de42_464e_a85a_83b1e0beb680  Port=9
  Add : Sum  Inputs=+++
  Convert to signed for subtraction : DataTypeConversion  RequirementInfo={} %GIDa_cb4dee5a_bff4_4ea7_9054_2c98110a9e9e  OutDataTypeStr=uint8
  Convert to signed for subtraction1 : DataTypeConversion  RequirementInfo={} %GIDa_ed795343_2e36_4503_9328_b45015374746  OutDataTypeStr=uint8
  Convert to signed for subtraction2 : DataTypeConversion  RequirementInfo={} %GIDa_f8af208a_0ee9_406e_8c03_b01738b03c2b  OutDataTypeStr=uint8
  Copyright1 : Subsystem  Description=|  RequirementInfo={} %GIDa_319df1af_001c_4cc4_b3eb_37fecdfa180d  mask(Copyright Information){none=on}
      | Copyright info block.                                               
      |                                                                     
      | Place copyright information at the top of every subsystem in design.
      mask prompts: none "No parameters"
      mask help: Place copyright information at the top of every subsystem in design.
      mask Display:
      | NxtrConf = 'Nexteer Confidential';
      | 
      | sys = bdroot; %handle for the current model ("system")
      | first = get_param(sys,'Created');
      | if(isempty(first))
      |     first = datestr(now,'yyyy');
      | else
      |     first = first(end-3:end);  %year is last four digits
      | end
      | 
      | last = get_param(sys,'LastModifiedDate');
      | if isempty(last)
      |     last = datestr(now,'yyyy');
      | else
      |     last = last(end-3:end);
      | end
      | 
      | if strcmp(first,last)
      |     fprintf('%s\nCopyright  %s Nexteer',NxtrConf,first);
      | else
      |     fprintf('%s\n%s%s-%s Nexteer',NxtrConf,char(169),first,last);
      | end
  Logical Operator1 : Logic  RequirementInfo={} %GIDa_4dbbbf24_014f_4a09_9636_be93a26e928f  Inputs=3  AllPortsSameDT=off  OutDataTypeStr=boolean
  Logical Operator2 : Logic  RequirementInfo={} %GIDa_1ed81b5b_8fad_4b26_8862_02a3d04d536c  Inputs=3  AllPortsSameDT=off  OutDataTypeStr=boolean
  Logical Operator4 : Logic  RequirementInfo={} %GIDa_f37b6da1_82d6_42d0_9feb_3380b34597c0  Inputs=3  AllPortsSameDT=off  OutDataTypeStr=boolean
  MOTAGACORRLNST_CNT_U08 : Constant  Value=MOTAGACORRLNST_CNT_U08
  MOTAGACORRLNST_CNT_U1 : Constant  Value=MOTAGBCORRLNST_CNT_U08
  MOTAGACORRLNST_CNT_U2 : Constant  Value=MOTAGCCORRLNST_CNT_U08
  Product : Product
  Product1 : Product
  Product2 : Product
  MotAgMeclCorrlnSt : Outport  RequirementInfo={} %GIDa_63e9bd03_806d_4347_a053_4557326ebccb
  wires:
  In1/1 -> Logical Operator1/1
  In2/1 -> Logical Operator1/2
  In3/1 -> Logical Operator1/3
  In4/1 -> Logical Operator4/1
  In5/1 -> Logical Operator4/2
  In6/1 -> Logical Operator4/3
  In7/1 -> Logical Operator2/1
  In8/1 -> Logical Operator2/2
  In9/1 -> Logical Operator2/3
  Logical Operator1/1 -> Convert to signed for subtraction/1
  Convert to signed for subtraction/1 -> Product/1
  MOTAGACORRLNST_CNT_U08/1 -> Product/2
  Logical Operator4/1 -> Convert to signed for subtraction1/1
  Convert to signed for subtraction1/1 -> Product1/1
  MOTAGACORRLNST_CNT_U1/1 -> Product1/2
  Logical Operator2/1 -> Convert to signed for subtraction2/1
  Convert to signed for subtraction2/1 -> Product2/1
  MOTAGACORRLNST_CNT_U2/1 -> Product2/2
  Product/1 -> Add/1
  Product1/1 -> Add/2
  Product2/1 -> Add/3
  Add/1 -> MotAgMeclCorrlnSt/1

== system ES249A_MotAgCorrln/MotAgCorrln/MotAgCorrlnPer1/Copyright1 ==

== system ES249A_MotAgCorrln/MotAgCorrln/MotAgCorrlnPer1/Fail Action  ==
  Action Port : ActionPort  ActionType=else
  Constant : Constant  Value=0  OutDataTypeStr=uint8
      settings: AttributesFormatString=%<OutDataTypeStr>
  Copyright1 : Subsystem  Description=|  mask(Copyright Information){none=on}
      | Copyright info block.                                               
      |                                                                     
      | Place copyright information at the top of every subsystem in design.
      mask prompts: none "No parameters"
      mask help: Place copyright information at the top of every subsystem in design.
      mask Display:
      | NxtrConf = 'Nexteer Confidential';
      | 
      | sys = bdroot; %handle for the current model ("system")
      | first = get_param(sys,'Created');
      | if(isempty(first))
      |     first = datestr(now,'yyyy');
      | else
      |     first = first(end-3:end);  %year is last four digits
      | end
      | 
      | last = get_param(sys,'LastModifiedDate');
      | if isempty(last)
      |     last = datestr(now,'yyyy');
      | else
      |     last = last(end-3:end);
      | end
      | 
      | if strcmp(first,last)
      |     fprintf('%s\nCopyright  %s Nexteer',NxtrConf,first);
      | else
      |     fprintf('%s\n%s%s-%s Nexteer',NxtrConf,char(169),first,last);
      | end
  MotAgMeclIdptSig : Outport  OutDataTypeStr=uint8
  wires:
  Constant/1 -> MotAgMeclIdptSig/1

== system ES249A_MotAgCorrln/MotAgCorrln/MotAgCorrlnPer1/FltInj_u08  ==
  note: This block requires no modification by FDD author.
      |
      | This block does not actually simulate any fault injection.  It is simply a pass-thru.
      |
      | The Constant port (#2) simply terminates its signal, but we are trying to force the FDD author
      | to properly use the FltInjectionLocType enumeration in FDD model.
  note: EA4.x Fault Injection
  Signal_In : Inport
  Constant : Inport  Port=2
  Copyright1 : Subsystem  Description=|  RequirementInfo={} %GIDa_0eace49f_b789_449d_b1ad_5a467ed07a04  mask(Copyright Information){none=on}
      | Copyright info block.                                               
      |                                                                     
      | Place copyright information at the top of every subsystem in design.
      mask prompts: none "No parameters"
      mask help: Place copyright information at the top of every subsystem in design.
      mask Display:
      | NxtrConf = 'Nexteer Confidential';
      | 
      | sys = bdroot; %handle for the current model ("system")
      | first = get_param(sys,'Created');
      | if(isempty(first))
      |     first = datestr(now,'yyyy');
      | else
      |     first = first(end-3:end);  %year is last four digits
      | end
      | 
      | last = get_param(sys,'LastModifiedDate');
      | if isempty(last)
      |     last = datestr(now,'yyyy');
      | else
      |     last = last(end-3:end);
      | end
      | 
      | if strcmp(first,last)
      |     fprintf('%s\nCopyright  %s Nexteer',NxtrConf,first);
      | else
      |     fprintf('%s\n%s%s-%s Nexteer',NxtrConf,char(169),first,last);
      | end
  Terminator : Terminator
  Signal_Out : Outport
  wires:
  Signal_In/1 -> Signal_Out/1
  Constant/1 -> Terminator/1

== system ES249A_MotAgCorrln/MotAgCorrln/MotAgCorrlnPer1/GetNtcQlfrSts 0x080  ==
  note: Enumeration of SigQlfr1
      |         SIGQLFR_NORES   (0)
      |         SIGQLFR_PASSD    (1)
      |         SIGQLFR_FAILD      (2)
  NtcNr : Inport
  CopyRight2 : Subsystem  Description=|  mask(Copyright Information){none=on}
      | Copyright info block.                                               
      |                                                                     
      | Place copyright information at the top of every subsystem in design.
      mask prompts: none "No parameters"
      mask help: Place copyright information at the top of every subsystem in design.
      mask Display:
      | NxtrConf = 'Nexteer Confidential';
      | 
      | sys = bdroot; %handle for the current model ("system")
      | first = get_param(sys,'Created');
      | first = first(end-3:end);  %year is last four digits
      | 
      | last = get_param(sys,'LastModifiedDate');
      | if isempty(last)
      |     last = datestr(now,'yyyy');
      | else
      |     last = last(end-3:end);
      | end
      | 
      | if strcmp(first,last)
      |     fprintf('%s -- Copyright %s Nexteer',NxtrConf,first)
      | else
      |     fprintf('%s -- %s%s- %s Nexteer',NxtrConf,char(169),first,last)
      | end
  Data Store Read5 : DataStoreRead  DataStoreName=NTC080Qlfr
  Data Type Conversion : DataTypeConversion  OutDataTypeStr=uint8
  EOK : Constant  OutDataTypeStr=uint8
  Terminator : Terminator
  Return : Outport  InitialOutput=1
  NtcQlfrSts : Outport  Port=2
  wires:
  Data Store Read5/1 -> Data Type Conversion/1
  EOK/1 -> Return/1
  NtcNr/1 -> Terminator/1
  Data Type Conversion/1 -> NtcQlfrSts/1

== system ES249A_MotAgCorrln/MotAgCorrln/MotAgCorrlnPer1/GetNtcQlfrSts 0x081 ==
  note: Enumeration of SigQlfr1
      |         SIGQLFR_NORES   (0)
      |         SIGQLFR_PASSD    (1)
      |         SIGQLFR_FAILD      (2)
  NtcNr : Inport
  CopyRight2 : Subsystem  Description=|  mask(Copyright Information){none=on}
      | Copyright info block.                                               
      |                                                                     
      | Place copyright information at the top of every subsystem in design.
      mask prompts: none "No parameters"
      mask help: Place copyright information at the top of every subsystem in design.
      mask Display:
      | NxtrConf = 'Nexteer Confidential';
      | 
      | sys = bdroot; %handle for the current model ("system")
      | first = get_param(sys,'Created');
      | first = first(end-3:end);  %year is last four digits
      | 
      | last = get_param(sys,'LastModifiedDate');
      | if isempty(last)
      |     last = datestr(now,'yyyy');
      | else
      |     last = last(end-3:end);
      | end
      | 
      | if strcmp(first,last)
      |     fprintf('%s -- Copyright %s Nexteer',NxtrConf,first)
      | else
      |     fprintf('%s -- %s%s- %s Nexteer',NxtrConf,char(169),first,last)
      | end
  Data Store Read5 : DataStoreRead  DataStoreName=NTC081Qlfr
  Data Type Conversion : DataTypeConversion  OutDataTypeStr=uint8
  EOK : Constant  OutDataTypeStr=uint8
  Terminator : Terminator
  Return : Outport  InitialOutput=1
  NtcQlfrSts : Outport  Port=2
  wires:
  Data Store Read5/1 -> Data Type Conversion/1
  EOK/1 -> Return/1
  NtcNr/1 -> Terminator/1
  Data Type Conversion/1 -> NtcQlfrSts/1

== system ES249A_MotAgCorrln/MotAgCorrln/MotAgCorrlnPer1/GetNtcQlfrSts 0x082 ==
  note: Enumeration of SigQlfr1
      |         SIGQLFR_NORES   (0)
      |         SIGQLFR_PASSD    (1)
      |         SIGQLFR_FAILD      (2)
  NtcNr : Inport
  CopyRight2 : Subsystem  Description=|  mask(Copyright Information){none=on}
      | Copyright info block.                                               
      |                                                                     
      | Place copyright information at the top of every subsystem in design.
      mask prompts: none "No parameters"
      mask help: Place copyright information at the top of every subsystem in design.
      mask Display:
      | NxtrConf = 'Nexteer Confidential';
      | 
      | sys = bdroot; %handle for the current model ("system")
      | first = get_param(sys,'Created');
      | first = first(end-3:end);  %year is last four digits
      | 
      | last = get_param(sys,'LastModifiedDate');
      | if isempty(last)
      |     last = datestr(now,'yyyy');
      | else
      |     last = last(end-3:end);
      | end
      | 
      | if strcmp(first,last)
      |     fprintf('%s -- Copyright %s Nexteer',NxtrConf,first)
      | else
      |     fprintf('%s -- %s%s- %s Nexteer',NxtrConf,char(169),first,last)
      | end
  Data Store Read5 : DataStoreRead  DataStoreName=NTC082Qlfr
  Data Type Conversion : DataTypeConversion  OutDataTypeStr=uint8
  EOK : Constant  OutDataTypeStr=uint8
  Terminator : Terminator
  Return : Outport  InitialOutput=1
  NtcQlfrSts : Outport  Port=2
  wires:
  Data Store Read5/1 -> Data Type Conversion/1
  EOK/1 -> Return/1
  NtcNr/1 -> Terminator/1
  Data Type Conversion/1 -> NtcQlfrSts/1
